simulink model "twintrackSimulinkTest"  (R2023b)
settings: Solver=ode45  StartTime=0.0  StopTime=140  MaxStep=0.01  RelTol=1e-8
libraries: simulink_extras x1, simulink x1
settings Model: PacingRate=9  Creator=eforce  LastModifiedBy=cigla
settings DebuggingCC: UnconnectedInputMsg=warning  UnconnectedOutputMsg=warning  UnconnectedLineMsg=warning
settings ModelReferenceCC: EnableRefExpFcnMdlSchedulingChecks=on
settings RTWCC: DLArmComputeVersion=19.05

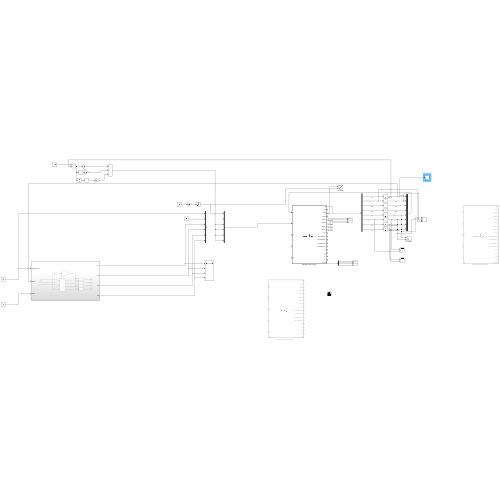
[thumbnail: Simulink's stored preview of the top-level diagram]
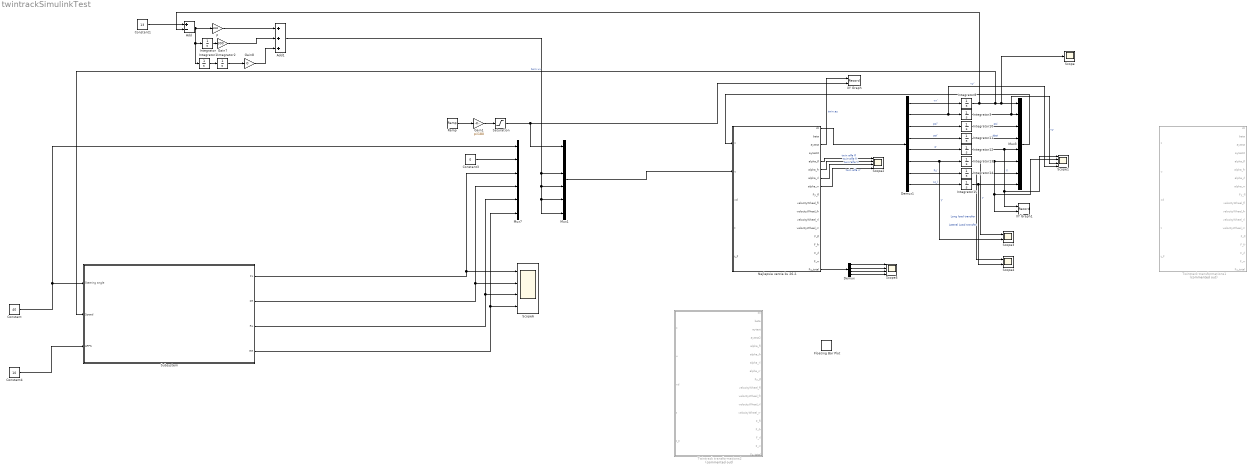
== system twintrackSimulinkTest ==
  Add : Sum  Inputs=+-
  Add1 : Sum  Inputs=+++
  Constant : Constant  Value=40
  Constant1 : Constant  Value=13
  Constant3 : Constant  Value=0
  Constant4 : Constant  Value=10
  Demux : Demux
  Demux1 : Demux  Outputs=8
  Floating Bar Plot : simulink_extras/Additional Sinks/Floating Bar Plot  yLim="[-100 100  -100 100  -100 100  -100 100  -5 5  -5 5  -5 5  -5 5  -5 5  -5 5  -5 5]"
  Gain1 : Gain  Gain=pi/180
  Gain7 : Gain  Gain=300
  Gain8 : Gain  Gain=0
  Integrator{,1..2,8,10..15} (10 alike) : Integrator
  Integrator3 : Integrator  ZeroCross=off
  Mux1 : Mux  Inputs=6
  Mux3 : Mux  Inputs=8
  Mux7 : Mux  Inputs=6
  Najlepsia verzia ku 26.2. : MATLAB Function  TreatAsAtomicUnit=on
  P : Gain  Gain=1000
  Ramp : simulink/Sources/Ramp  slope=0.1  start=10  InitialOutput=0
  Saturation : Saturate  UpperLimit=25  LowerLimit=-25
  Scope : Scope
  Scope{1..2,5..6} (4 alike) : Scope  NumInputPorts=4
  Scope3 : Scope  NumInputPorts=2
  Scope4 : Scope  NumInputPorts=2
  Subsystem : Subsystem
  Twintrack transformations1 : MATLAB Function  Commented=on  TreatAsAtomicUnit=on
  Twintrack transformations2 : MATLAB Function  Commented=on  TreatAsAtomicUnit=on
  XY Graph : Record  FileSettingsInternal="{\"entries\":[{\"content\":{\"excelSettings\":{\"content\":{},\"type\":\"Streamout.ExcelSettings\"}},\"type\":\"Streamout.FileSettingStorage\",\"uuid\":\"\"}],\"packageUris\":[\"http:\\/\\/schema.mathworks.com\\/mf0\\/streamout_blocks\\/R2020a\"],\"version\":\"1.0\"}"  Layout=[1 1]  SignalsInternal="{\"entries\":[{\"content\":{\"signals\":[{\"content\":{\"blockPath\":[],\"dimensions\":[1],\"domain\":\"\",\"lineColor\":\"#edb120\",\"plots\":[1],\"port\":1,\"sid\":[\"\"],\"signalID\":3270,\"signalName\":\"twin.ay\"},\"type\":\"RecordBlkView.Signal\",\"uuid\":\"\"},{\"content\":{\"blockPath\":[],\"dimensions\":[1],\"domain\":\"\",\"lineColor\":\"#7e2f8e\",\"plots\":[1],\"port\":2,\"sid\":[\"\"],\"signalID\":3274,\"signalName\":\"Saturation\"},\"type\":\"RecordBlkView.Signal\",\"uuid\":\"\"}]},\"type\":\"RecordBlkView.InputSignals\",\"uuid\":\"\"}],\"packageUris\":[\"http:\\/\\/schema.mathworks.com\\/mf0\\/streamout_blocks\\/R2020a\"],\"version\":\"1.0\"}"  VisualizationBindings="{\"xyplotplugin\":{\"info\":[{\"series\":[{\"bindingParametersList\":[{\"parameter\":\"X-Axis\",\"signalID\":3270,\"signalName\":\"twin.ay\"},{\"parameter\":\"Y-Axis\",\"signalID\":3274,\"signalName\":\"Saturation\"}],\"seriesID\":12474}],\"subplotID\":1}]}}"  CompatibilityTag=XY
  XY Graph1 : Record  FileSettingsInternal="{\"entries\":[{\"content\":{\"excelSettings\":{\"content\":{},\"type\":\"Streamout.ExcelSettings\"}},\"type\":\"Streamout.FileSettingStorage\",\"uuid\":\"\"}],\"packageUris\":[\"http:\\/\\/schema.mathworks.com\\/mf0\\/streamout_blocks\\/R2020a\"],\"version\":\"1.0\"}"  Layout=[1 1]  SignalsInternal="{\"entries\":[{\"content\":{\"signals\":[{\"content\":{\"blockPath\":[],\"dimensions\":[1],\"domain\":\"\",\"lineColor\":\"#77ac30\",\"plots\":[1],\"port\":1,\"sid\":[\"\"],\"signalID\":3278,\"signalName\":\"X\"},\"type\":\"RecordBlkView.Signal\",\"uuid\":\"\"},{\"content\":{\"blockPath\":[],\"dimensions\":[1],\"domain\":\"\",\"lineColor\":\"#4dbeee\",\"plots\":[1],\"port\":2,\"sid\":[\"\"],\"signalID\":3282,\"signalName\":\"Y\"},\"type\":\"RecordBlkView.Signal\",\"uuid\":\"\"}]},\"type\":\"RecordBlkView.InputSignals\",\"uuid\":\"\"}],\"packageUris\":[\"http:\\/\\/schema.mathworks.com\\/mf0\\/streamout_blocks\\/R2020a\"],\"version\":\"1.0\"}"  VisualizationBindings="{\"xyplotplugin\":{\"info\":[{\"series\":[{\"bindingParametersList\":[{\"parameter\":\"X-Axis\",\"signalID\":3278,\"signalName\":\"X\"},{\"parameter\":\"Y-Axis\",\"signalID\":3282,\"signalName\":\"Y\"}],\"seriesID\":46744}],\"subplotID\":1}]}}"  CompatibilityTag=XY
  wires:
  Constant3/1 -> Mux7/2
  Constant1/1 -> Add/1
  Integrator2/1 -> Gain8/1
  Integrator1/1 -> Integrator2/1
  Mux1/1 -> Najlepsia verzia ku 26.2./2(u)
  Gain7/1 -> Add1/2
  Gain8/1 -> Add1/3
  P/1 -> Add1/1
  Add/1 -> P/1, Integrator/1, Integrator1/1
  Integrator/1 -> Gain7/1
  Integrator8/1 -> Subsystem/2(Speed), Scope/1, Mux3/1, Add/2  "twin.vx"
  Demux1/4 -> Integrator11/1  "psi'"
  Integrator13/1 -> Scope3/1, XY Graph1/2, Scope1/2, Mux3/6  "Y"
  Integrator10/1 -> Mux3/3  "psi"
  Demux1/1 -> Integrator8/1  "vx'"
  Demux1/6 -> Scope3/2, Integrator13/1  "Y'"
  Integrator3/1 -> Scope1/3, Mux3/2  "vy"
  Demux1/7 -> Integrator14/1  "Fz'"
  Demux1/3 -> Integrator10/1  "psi''"
  Demux1/2 -> Scope1/4, Integrator3/1  "vy'"
  Integrator11/1 -> Mux3/4  "dpsi"
  Demux1/5 -> Integrator12/1  "X'"
  Integrator12/1 -> XY Graph1/1, Scope1/1, Mux3/5  "X"
  Demux1/8 -> Integrator15/1  "Lt_l"
  Integrator15/1 -> Scope4/2, Mux3/8  "Lateral Load transfer"
  Integrator14/1 -> Scope4/1, Mux3/7  "Long load transfer"
  Najlepsia verzia ku 26.2./1(dz) -> Demux1/1
  Najlepsia verzia ku 26.2./3(aytest) -> XY Graph/1  "twin.ay"
  Mux3/1 -> Najlepsia verzia ku 26.2./1(z)
  Saturation/1 -> XY Graph/2, Mux1/1
  Najlepsia verzia ku 26.2./18(Fz_total) -> Demux/1
  Demux/1 -> Scope5/1
  Demux/2 -> Scope5/2
  Demux/3 -> Scope5/3
  Demux/4 -> Scope5/4
  Constant/1 -> Mux7/1, Subsystem/1(Steering angle)
  Constant4/1 -> Subsystem/3(APPS)
  Subsystem/1(FL) -> Mux7/3, Scope6/1
  Subsystem/2(FR) -> Scope6/2, Mux7/4
  Subsystem/3(RL) -> Mux7/5, Scope6/3
  Subsystem/4(RR) -> Mux7/6, Scope6/4
  Add1/1 -> Mux1/6, Mux1/5, Mux1/4, Mux1/3
  Ramp/1 -> Gain1/1
  Gain1/1 -> Saturation/1
  Najlepsia verzia ku 26.2./5(alpha_fl) -> Scope2/1  "twin alfa fl"
  Najlepsia verzia ku 26.2./6(alpha_fr) -> Scope2/2  "twin alfa fr"
  Najlepsia verzia ku 26.2./7(alpha_rl) -> Scope2/3  "twin alfa rl"
  Najlepsia verzia ku 26.2./8(alpha_rr) -> Scope2/4  "twin alfa rr"

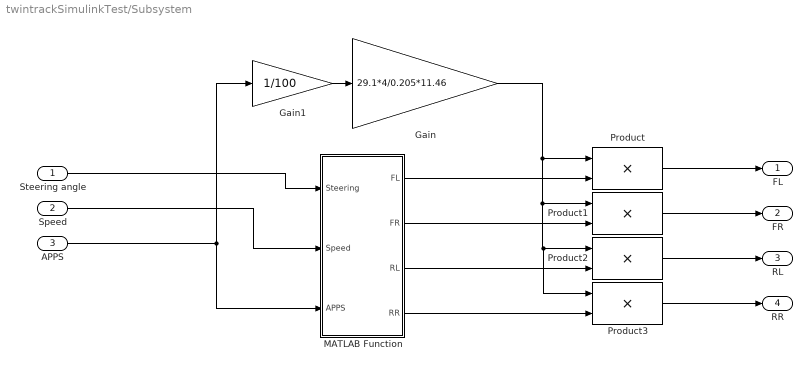
== system twintrackSimulinkTest/Subsystem ==
  Steering angle : Inport
  Speed : Inport  Port=2
  APPS : Inport  Port=3
  Gain : Gain  Gain=29.1*4/0.205*11.46
  Gain1 : Gain  Gain=1/100
  MATLAB Function : MATLAB Function  TreatAsAtomicUnit=on
  Product{,1..3} (4 alike) : Product
  FL : Outport
  FR : Outport  Port=2
  RL : Outport  Port=3
  RR : Outport  Port=4
  wires:
  Steering angle/1 -> MATLAB Function/1(Steering)
  Speed/1 -> MATLAB Function/2(Speed)
  APPS/1 -> Gain1/1, MATLAB Function/3(APPS)
  Gain1/1 -> Gain/1
  MATLAB Function/1(FL) -> Product/2
  Gain/1 -> Product3/1, Product2/1, Product1/1, Product/1
  MATLAB Function/2(FR) -> Product1/2
  MATLAB Function/3(RL) -> Product2/2
  MATLAB Function/4(RR) -> Product3/2
  Product/1 -> FL/1
  Product1/1 -> FR/1
  Product2/1 -> RL/1
  Product3/1 -> RR/1

== matlab function twintrackSimulinkTest/Twintrack transformations2 ==
  data: z input size=8; u input size=6; dz output size=8; xd input; t input; t_F input; beta output; aytest output; aytest2 output; alpha_fl output; alpha_fr output; alpha_rl output; alpha_rr output; Fy_fl output; velocityWheel_fl output size=[1 3]; velocityWheel_fr output size=[1 3]; velocityWheel_rl output size=[1 3]; velocityWheel_rr output size=[1 3]; F_fl output size=[1 2]; F_fr output size=[1 2]; F_rl output size=[1 2]; F_rr output size=[1 2]; Fz_total output size=[1 4]
function [dz, beta, aytest, aytest2,alpha_fl,alpha_fr,alpha_rl,alpha_rr,Fy_fl,velocityWheel_fl,velocityWheel_fr,velocityWheel_rl,velocityWheel_rr,F_fl,F_fr,F_rl,F_rr,Fz_total]= twinRaceCar_time_ODE(z, u, xd, t, t_F)
% z = [vx; vy; psi; dpsidt; X; Y], vx-longitudinal velocity, vy-lateral velocity, psi-angular position of the car with respect to the inertial frame, X and Y are coordinates of the car in the inertial frame
% u = [delta_f; delta_r; Ff; Fr], delta_f - steering angle of the front wheel, delta_r - steering angle of the rear wheel (NOT IMPLEMENTED YET), Ff - force acting on the front wheel in the longitudinal direction, Fr - force acting on the rear wheel in the longitudinal direction
% car - structure containing parameters of the car model




%%%%%%%%%%%%%%%%%%%% Car parameters %%%%%%%%%%%%%%%%%%%%
tracks       = 2;
m            = 280;                      % weight of the car [kg]
Izz          = 100;                      % moment of inertia [kg m^2]
wheelbase    = 1.530;%1.575;                    % distance between the front and rear axles [m];
track        = 1*1.2;                      % distance between right and left wheel
COGr         = 0.4876;                       % COG distribution 0-1 scale on rear
COG          = wheelbase*(COGr); % distance of Center Of Gravity (COG) from the front axle [m];
l_f          = COG;                  % distance of the front axle form the COG [m];
l_r          = wheelbase - COG;  % distance of the rear axle form the COG [m];
COGz         = 0.3;                      % height of COG from ground
wheelradius  = 0.205;                    % radius of the wheels [m]
steeringAngle_max = 20/180*pi;           % Maximum allowed steering angle
steeringAngle_maxRate = 400/180*pi;      % Maximum allowed steering angle [rad/s]
%% Motor parameters
Mf_max       = 29.1 * 2/tracks * 11.46;         % maximum torque generated by a motor on the front axle [Nm]
Mf_slewRate  = 16000;                      % maximum slew rate of the generated torque on the rear axle [Nm/s]0.5 je ca 1000/s idk preco
Mf_jerk       = 800;                           % 1000 bolo cca okay
Mr_max       = 29.1 * 2/tracks * 11.46;         % maximum torque generated by a motor on the rear axle [Nm]
Mr_slewRate  = 100;                      % maximum slew rate of the generated torque on the rear axle [Nm/s]
Yt_max       = (Mf_max/wheelradius + Mr_max/wheelradius)*track;                    % maximum Yaw moment
PwrMax       = 80000;
PwrMin       = -40000;
maxSpeed     = 40;                        %m/sftire


%% Tire and suspension parameters
E = 0.23;
D = 1.2;
B = 0.2;
C = 1.3;


Sus_t = 10;                          % suspension time constant for 1st order system
tire_fxFactor = 1.5 ;                 % max Fx = Fz * tire_fxFactor
tire_fyFactor = 1.3;                 % max Fy = Fz * tire_fyFactor
%ftire = @(alph, Fz, p)(alph/pi*180)* Fz * tire_stifness ; %
ftire = @(alph,Fz, p)  Fz* D*sin(C*atan(B*(alph/pi*180)  - E*atan(B*(alph/pi*180))));
ftire = @(alph, Fz)(alph./pi.*180)./3.* Fz .* tire_fyFactor ; %
%ftire = @(alph, Fz) min((alph./pi.*180)./15.* Fz .* tire_fyFactor ,(deg2rad(15)./pi.*180)./15.* Fz.* tire_fyFactor ) ; %
%% Aerodynamics parameters
CL  = -4.15;
CD  = 1.55;
A   = 1;
COP = 0.5;    % Center of pressure on rear ratio
wingLength_f = 0.9;

%% environment parameters
g = 9.81;
airDensity = 1.225;


    Ft = u;

% Extract the controls from F
delta_f   = Ft(1);
delta_r   = Ft(2);
Fx_fl     = Ft(3);
Fx_fr     = Ft(4);
Fx_rl     = Ft(5);
Fx_rr     = Ft(6);


%% Extract the states from z
v_x  = z(1);
v_y  = z(2);
psi  = z(3);
dpsi = z(4);
X    = z(5);
Y    = z(6);
Fz   = z(7);
Ltl  = z(8);
%% Compute the slip angles
%% Compute the slip angles
%% initialize matrices, origin of car is in COG
v = [v_x v_y 0];
dpsiv = [ 0 0 dpsi];
pos_fr = [  l_f  -track/2 0];
pos_fl = [  l_f   track/2 0];
pos_rr = [ -l_r -track/2 0];
pos_rl = [ -l_r  track/2 0];

%% Calculate vectors at uprights
velocityUpright_fl = v + cross(dpsiv,pos_fl);
velocityUpright_fr = v + cross(dpsiv,pos_fr);
velocityUpright_rl = v + cross(dpsiv,pos_rl);
velocityUpright_rr = v + cross(dpsiv,pos_rr);

%% Define Rotation matrices
rotate_f = [
    cos(delta_f) -sin(delta_f) 0
    sin(delta_f) cos(delta_f)  0
    0            0             0
    ];
rotate_r = [
    cos(delta_r) -sin(delta_r) 0
    sin(delta_r) cos(delta_r)  0
    0            0             0
    ];

%% Calculate wheel velocity in wheel frames
velocityWheel_fl = velocityUpright_fl * rotate_f;
velocityWheel_fr = velocityUpright_fr * rotate_f;
velocityWheel_rl = velocityUpright_rl * rotate_r;
velocityWheel_rr = velocityUpright_rr * rotate_r;


%% Calculate alphas
alpha_fl = -atan2(velocityWheel_fl(2),velocityWheel_fl(1));
alpha_fr = -atan2(velocityWheel_fr(2),velocityWheel_fr(1));
alpha_rl = -atan2(velocityWheel_rl(2),velocityWheel_rl(1));
alpha_rr = -atan2(velocityWheel_rr(2),velocityWheel_rr(1));


%% Compute the forces acting on the wheels
Fz_aero = 0.5*airDensity*CL*A*v_x.^2;
Fz_f = m/2*(1-COGr) * g - Fz/2 - Fz_aero/2 * (1-COP);
Fz_r = m/2*(COGr)   * g + Fz/2 - Fz_aero/2 * COP;

Fz_fl = m/2*(1-COGr) * g - Fz/2 - Fz_aero/2 * (1-COP) + Ltl/2;
Fz_fr = m/2*(1-COGr) * g - Fz/2 - Fz_aero/2 * (1-COP) - Ltl/2;
Fz_rl = m/2*(COGr)   * g + Fz/2 - Fz_aero/2 * COP + Ltl/2;
Fz_rr = m/2*(COGr)   * g + Fz/2 - Fz_aero/2 * COP - Ltl/2;

Fy_fl = ftire(alpha_fl,Fz_fl);
Fy_fr = ftire(alpha_fr,Fz_fr);
Fy_rl = ftire(alpha_rl,Fz_rl);
Fy_rr = ftire(alpha_rr,Fz_rr);

%% Projection of forces from steered wheels to uprights
projection_f = [
    cos(delta_f)      sin(delta_f)
    -sin(delta_f)     cos(delta_f)   
    ];
projection_r = [
    cos(delta_r)      sin(delta_r)
    -sin(delta_r)     cos(delta_r)   
    ];
%% Forces acting on uprights
F_fl = [Fx_fl Fy_fl] * projection_f;
F_fr = [Fx_fr Fy_fr] * projection_f;
F_rl = [Fx_rl Fy_rl] * projection_r;
F_rr = [Fx_rr Fy_rr] * projection_r;

F_drag = 0.5*airDensity*CD*A*v_x^2;
% Compute quantities need for the change of the position in the inertial frame
v = sqrt(v_x^2 + v_y^2);
beta = atan2(v_y, v_x);

M = (F_fr(1) + F_rr(1) - F_fl(1) - F_rl(1))*track/2 +... % Forward forces create Moment
    (F_fr(2) + F_fl(2)) * l_f...                         % Lateral forces from front tires
   -(F_rr(2) + F_rl(2)) * l_r;                          % Lateral forces from rear tires

Fx = F_fr(1) + F_rr(1) + F_fl(1) + F_rl(1)- F_drag;         % Longitudinal force from wheels and drag
Fy = F_fr(2) + F_rr(2) + F_fl(2) + F_rl(2);                  % Lateral force
aytest = Fy/m;
aytest2 = -dpsi*v_x;
Fz_total = [Fz_fl Fz_fr Fz_rl Fz_rr];
%dvx = 1/m  * (F_rx*cos(delta_r) - F_ry*sin(delta_r) + F_fx*cos(delta_f) - F_fy*sin(delta_f) - 0.5*airDensity*CD*A*v_x^2) + dpsi*v_y;
dz = [... 
Fx/m  + dpsi*v_y                                                                                                                      % v_x/dt
Fy/m  - dpsi*v_x                      % v_y/dt  
dpsi;                                                                                                                         % psi/dt
M/Izz   % dpsi
v*cos(psi + beta);                                                                                                            % X/dt
v*sin(psi + beta);                                                                                                            % Y/dt
((Fx/m + dpsi*v_y) *COGz/wheelbase*m-Fz)/Sus_t;                                                                              %Fz/dt  
((- dpsi*v_x) *COGz/track*m-Ltl)/Sus_t;
];

M=4;
end

== matlab function twintrackSimulinkTest/Twintrack transformations1 ==
  data: z input size=8; u input size=6; dz output size=8; xd input; t input; t_F input; beta output; aytest output; aytest2 output; alpha_fl output; alpha_fr output; alpha_rl output; alpha_rr output; Fy_fl output; velocityWheel_fl output size=[1 3]; velocityWheel_fr output size=[1 3]; velocityWheel_rl output size=[1 3]; velocityWheel_rr output size=[1 3]; F_fl output size=[1 2]; F_fr output size=[1 2]; F_rl output size=[1 2]; F_rr output size=[1 2]; Fz_total output size=[1 4]
function [dz, beta, aytest, aytest2,alpha_fl,alpha_fr,alpha_rl,alpha_rr,Fy_fl,velocityWheel_fl,velocityWheel_fr,velocityWheel_rl,velocityWheel_rr,F_fl,F_fr,F_rl,F_rr,Fz_total]= twinRaceCar_time_ODE(z, u, xd, t, t_F)
% z = [vx; vy; psi; dpsidt; X; Y], vx-longitudinal velocity, vy-lateral velocity, psi-angular position of the car with respect to the inertial frame, X and Y are coordinates of the car in the inertial frame
% u = [delta_f; delta_r; Ff; Fr], delta_f - steering angle of the front wheel, delta_r - steering angle of the rear wheel (NOT IMPLEMENTED YET), Ff - force acting on the front wheel in the longitudinal direction, Fr - force acting on the rear wheel in the longitudinal direction
% car - structure containing parameters of the car model




%%%%%%%%%%%%%%%%%%%% Car parameters %%%%%%%%%%%%%%%%%%%%
tracks       = 2;
m            = 280;                      % weight of the car [kg]
Izz          = 100;                      % moment of inertia [kg m^2]
wheelbase    = 1.530;%1.575;                    % distance between the front and rear axles [m];
track        = 1*1.2;                      % distance between right and left wheel
COGr         = 0.4876;                       % COG distribution 0-1 scale on rear
COG          = wheelbase*(COGr); % distance of Center Of Gravity (COG) from the front axle [m];
l_f          = COG;                  % distance of the front axle form the COG [m];
l_r          = wheelbase - COG;  % distance of the rear axle form the COG [m];
COGz         = 0.3;                      % height of COG from ground
wheelradius  = 0.205;                    % radius of the wheels [m]
steeringAngle_max = 20/180*pi;           % Maximum allowed steering angle
steeringAngle_maxRate = 400/180*pi;      % Maximum allowed steering angle [rad/s]
%% Motor parameters
Mf_max       = 29.1 * 2/tracks * 11.46;         % maximum torque generated by a motor on the front axle [Nm]
Mf_slewRate  = 16000;                      % maximum slew rate of the generated torque on the rear axle [Nm/s]0.5 je ca 1000/s idk preco
Mf_jerk       = 800;                           % 1000 bolo cca okay
Mr_max       = 29.1 * 2/tracks * 11.46;         % maximum torque generated by a motor on the rear axle [Nm]
Mr_slewRate  = 100;                      % maximum slew rate of the generated torque on the rear axle [Nm/s]
Yt_max       = (Mf_max/wheelradius + Mr_max/wheelradius)*track;                    % maximum Yaw moment
PwrMax       = 80000;
PwrMin       = -40000;
maxSpeed     = 40;                        %m/sftire


%% Tire and suspension parameters
E = 0.23;
D = 1.2;
B = 0.2;
C = 1.3;


Sus_t = 10;                          % suspension time constant for 1st order system
tire_fxFactor = 1.5 ;                 % max Fx = Fz * tire_fxFactor
tire_fyFactor = 1.3;                 % max Fy = Fz * tire_fyFactor
%ftire = @(alph, Fz, p)(alph/pi*180)* Fz * tire_stifness ; %
ftire = @(alph,Fz, p)  Fz* D*sin(C*atan(B*(alph/pi*180)  - E*atan(B*(alph/pi*180))));
%ftire = @(alph, Fz)(alph./pi.*180)./3.* Fz .* tire_fyFactor ; %
%ftire = @(alph, Fz) min((alph./pi.*180)./15.* Fz .* tire_fyFactor ,(deg2rad(15)./pi.*180)./15.* Fz.* tire_fyFactor ) ; %
%% Aerodynamics parameters
CL  = -4.15;
CD  = 1.55;
A   = 1;
COP = 0.5;    % Center of pressure on rear ratio
wingLength_f = 0.9;

%% environment parameters
g = 9.81;
airDensity = 1.225;


    Ft = u;

% Extract the controls from F
delta_f   = Ft(1);
delta_r   = Ft(2);
Fx_fl     = Ft(3);
Fx_fr     = Ft(4);
Fx_rl     = Ft(5);
Fx_rr     = Ft(6);


%% Extract the states from z
v_x  = z(1);
v_y  = z(2);
psi  = z(3);
dpsi = z(4);
X    = z(5);
Y    = z(6);
Fz   = z(7);
Ltl  = z(8);
%% Compute the slip angles
%% Compute the slip angles
%% initialize matrices, origin of car is in COG
v = [v_x v_y 0];
dpsiv = [ 0 0 dpsi];
pos_fr = [  l_f  -track/2 0];
pos_fl = [  l_f   track/2 0];
pos_rr = [ -l_r -track/2 0];
pos_rl = [ -l_r  track/2 0];

%% Calculate vectors at uprights
velocityUpright_fl = v + cross(dpsiv,pos_fl);
velocityUpright_fr = v + cross(dpsiv,pos_fr);
velocityUpright_rl = v + cross(dpsiv,pos_rl);
velocityUpright_rr = v + cross(dpsiv,pos_rr);

%% Define Rotation matrices
rotate_f = [
    cos(delta_f) -sin(delta_f) 0
    sin(delta_f) cos(delta_f)  0
    0            0             0
    ];
rotate_r = [
    cos(delta_r) -sin(delta_r) 0
    sin(delta_r) cos(delta_r)  0
    0            0             0
    ];

%% Calculate wheel velocity in wheel frames
velocityWheel_fl = velocityUpright_fl * rotate_f;
velocityWheel_fr = velocityUpright_fr * rotate_f;
velocityWheel_rl = velocityUpright_rl * rotate_r;
velocityWheel_rr = velocityUpright_rr * rotate_r;


%% Calculate alphas
alpha_fl = -atan2(velocityWheel_fl(2),velocityWheel_fl(1));
alpha_fr = -atan2(velocityWheel_fr(2),velocityWheel_fr(1));
alpha_rl = -atan2(velocityWheel_rl(2),velocityWheel_rl(1));
alpha_rr = -atan2(velocityWheel_rr(2),velocityWheel_rr(1));


%% Compute the forces acting on the wheels
Fz_aero = 0.5*airDensity*CL*A*v_x.^2;
Fz_f = m/2*(1-COGr) * g - Fz/2 - Fz_aero/2 * (1-COP);
Fz_r = m/2*(COGr)   * g + Fz/2 - Fz_aero/2 * COP;

Fz_fl = m/2*(1-COGr) * g - Fz/2 - Fz_aero/2 * (1-COP) + Ltl/2;
Fz_fr = m/2*(1-COGr) * g - Fz/2 - Fz_aero/2 * (1-COP) - Ltl/2;
Fz_rl = m/2*(COGr)   * g + Fz/2 - Fz_aero/2 * COP + Ltl/2;
Fz_rr = m/2*(COGr)   * g + Fz/2 - Fz_aero/2 * COP - Ltl/2;

Fz_total = [Fz_fl Fz_fr Fz_rl Fz_rr];

Fy_fl = ftire(alpha_fl,Fz_fl);
Fy_fr = ftire(alpha_fr,Fz_fr);
Fy_rl = ftire(alpha_rl,Fz_rl);
Fy_rr = ftire(alpha_rr,Fz_rr);

%% Projection of forces from steered wheels to uprights
projection_f = [
    cos(delta_f)      sin(delta_f)
    -sin(delta_f)     cos(delta_f)   
    ];

%projection_f = [
%    -cos(delta_f)      sin(delta_f)
%    sin(delta_f)     cos(delta_f)   
%    ];

projection_r = [
    cos(delta_r)      sin(delta_r)
    -sin(delta_r)     cos(delta_r)   
    ];
%% Forces acting on uprights
F_fl = [Fx_fl Fy_fl] * projection_f;
F_fr = [Fx_fr Fy_fr] * projection_f;
F_rl = [Fx_rl Fy_rl] * projection_r;
F_rr = [Fx_rr Fy_rr] * projection_r;

F_drag = 0.5*airDensity*CD*A*v_x^2;
% Compute quantities need for the change of the position in the inertial frame
v = sqrt(v_x^2 + v_y^2);
beta = atan2(v_y, v_x);

M = (F_fr(1) + F_rr(1) - F_fl(1) - F_rl(1))*track/2 +... % Forward forces create Moment
    (F_fr(2) + F_fl(2)) * l_f...                         % Lateral forces from front tires
   -(F_rr(2) + F_rl(2)) * l_r;                          % Lateral forces from rear tires

Fx = F_fr(1) + F_rr(1) + F_fl(1) + F_rl(1)- F_drag;         % Longitudinal force from wheels and drag
Fy = F_fr(2) + F_rr(2) + F_fl(2) + F_rl(2);                  % Lateral force

aytest = Fy/m;
aytest2 = -dpsi*v_x;

%dvx = 1/m  * (F_rx*cos(delta_r) - F_ry*sin(delta_r) + F_fx*cos(delta_f) - F_fy*sin(delta_f) - 0.5*airDensity*CD*A*v_x^2) + dpsi*v_y;
dz = [... 
Fx/m  + dpsi*v_y                                                                                                                      % v_x/dt
Fy/m  - dpsi*v_x                      % v_y/dt  
dpsi;                                                                                                                         % psi/dt
M/Izz   % dpsi
v*cos(psi + beta);                                                                                                            % X/dt
v*sin(psi + beta);                                                                                                            % Y/dt
((Fx/m + dpsi*v_y) *COGz/wheelbase*m-Fz)/Sus_t;                                                                              %Fz/dt  
((- dpsi*v_x) *COGz/track*m-Ltl)/Sus_t;
];

M=4;
end

== matlab function twintrackSimulinkTest/Subsystem/MATLAB Function ==
  data: Steering input; FL output; Speed input; APPS input; FR output; RL output; RR output
function [FL,FR,RL,RR] = fcn(Steering, Speed, APPS)

kL = 0.4;
k1 = 10;
kS = 0.75;

Steer_cal =Steering-50;
Mz = APPS*kL-Speed*(kL*APPS/33)+50+k1;
Ms = Steer_cal*kS-Speed*(kS*Steer_cal/33);



FL = 50-(Mz/2)+(Ms/2);
FR = 50-(Mz/2)-(Ms/2);

RL  =Mz/2+(Ms/2); 
RR  =(Mz/2)-(Ms/2);

== matlab function twintrackSimulinkTest/Najlepsia verzia ku 26.2. ==
  data: z input size=8; u input size=6; dz output size=8; xd input; t input; t_F input; beta output; aytest output; aytest2 output; alpha_fl output; alpha_fr output; alpha_rl output; alpha_rr output; Fy_fl output; velocityWheel_fl output size=[1 3]; velocityWheel_fr output size=[1 3]; velocityWheel_rl output size=[1 3]; velocityWheel_rr output size=[1 3]; F_fl output size=[1 2]; F_fr output size=[1 2]; F_rl output size=[1 2]; F_rr output size=[1 2]; Fz_total output size=[1 4]
function [dz, beta, aytest, aytest2,alpha_fl,alpha_fr,alpha_rl,alpha_rr,Fy_fl,velocityWheel_fl,velocityWheel_fr,velocityWheel_rl,velocityWheel_rr,F_fl,F_fr,F_rl,F_rr,Fz_total]= twinRaceCar_time_ODE(z, u, xd, t, t_F)
% z = [vx; vy; psi; dpsidt; X; Y], vx-longitudinal velocity, vy-lateral velocity, psi-angular position of the car with respect to the inertial frame, X and Y are coordinates of the car in the inertial frame
% u = [delta_f; delta_r; Ff; Fr], delta_f - steering angle of the front wheel, delta_r - steering angle of the rear wheel (NOT IMPLEMENTED YET), Ff - force acting on the front wheel in the longitudinal direction, Fr - force acting on the rear wheel in the longitudinal direction
% car - structure containing parameters of the car model




%%%%%%%%%%%%%%%%%%%% Car parameters %%%%%%%%%%%%%%%%%%%%
tracks       = 2;
m            = 280;                      % weight of the car [kg]
Izz          = 100;                      % moment of inertia [kg m^2]
wheelbase    = 1.530;%1.575;                    % distance between the front and rear axles [m];
track        = 1*1.2;                      % distance between right and left wheel
COGr         = 0.4876;                       % COG distribution 0-1 scale on rear
COG          = wheelbase*(COGr); % distance of Center Of Gravity (COG) from the front axle [m];
l_f          = COG;                  % distance of the front axle form the COG [m];
l_r          = wheelbase - COG;  % distance of the rear axle form the COG [m];
COGz         = 0.3;                      % height of COG from ground
wheelradius  = 0.205;                    % radius of the wheels [m]
steeringAngle_max = 20/180*pi;           % Maximum allowed steering angle
steeringAngle_maxRate = 400/180*pi;      % Maximum allowed steering angle [rad/s]
%% Motor parameters
Mf_max       = 29.1 * 2/tracks * 11.46;         % maximum torque generated by a motor on the front axle [Nm]
Mf_slewRate  = 16000;                      % maximum slew rate of the generated torque on the rear axle [Nm/s]0.5 je ca 1000/s idk preco
Mf_jerk       = 800;                           % 1000 bolo cca okay
Mr_max       = 29.1 * 2/tracks * 11.46;         % maximum torque generated by a motor on the rear axle [Nm]
Mr_slewRate  = 100;                      % maximum slew rate of the generated torque on the rear axle [Nm/s]
Yt_max       = (Mf_max/wheelradius + Mr_max/wheelradius)*track;                    % maximum Yaw moment
PwrMax       = 80000;
PwrMin       = -40000;
maxSpeed     = 40;                        %m/sftire


%% Tire and suspension parameters
E = 0.23;
D = 1.2;
B = 0.2;
C = 1.3;


Sus_t = 0.05;                          % suspension time constant for 1st order system
tire_fxFactor = 1.5 ;                 % max Fx = Fz * tire_fxFactor
tire_fyFactor = 1.3;                 % max Fy = Fz * tire_fyFactor
%ftire = @(alph, Fz, p)(alph/pi*180)* Fz * tire_stifness ; %
ftire = @(alph,Fz, p)  Fz* D*sin(C*atan(B*(alph/pi*180)  - E*atan(B*(alph/pi*180))));
ftire = @(alph, Fz)(alph./pi.*180)./3.* Fz .* tire_fyFactor ; %
%ftire = @(alph, Fz) min((alph./pi.*180)./15.* Fz .* tire_fyFactor ,(deg2rad(15)./pi.*180)./15.* Fz.* tire_fyFactor ) ; %
%% Aerodynamics parameters
CL  = -4.15;
CD  = 1.55;
A   = 1;
COP = 0.5;    % Center of pressure on rear ratio
wingLength_f = 0.9;

%% environment parameters
g = 9.81;
airDensity = 1.225;


    Ft = u;

% Extract the controls from F
delta_f   = Ft(1);
delta_r   = Ft(2);
Fx_fl     = Ft(3);
Fx_fr     = Ft(4);
Fx_rl     = Ft(5);
Fx_rr     = Ft(6);


%% Extract the states from z
v_x  = z(1);
v_y  = z(2);
psi  = z(3);
dpsi = z(4);
X    = z(5);
Y    = z(6);
Fz   = z(7);
Ltl  = z(8);
%% Compute the slip angles
%% Compute the slip angles
%% initialize matrices, origin of car is in COG
v = [v_x v_y 0];
dpsiv = [ 0 0 dpsi];
pos_fr = [  l_f  -track/2 0];
pos_fl = [  l_f   track/2 0];
pos_rr = [ -l_r -track/2 0];
pos_rl = [ -l_r  track/2 0];

%% Calculate vectors at uprights
velocityUpright_fl = v + cross(dpsiv,pos_fl);
velocityUpright_fr = v + cross(dpsiv,pos_fr);
velocityUpright_rl = v + cross(dpsiv,pos_rl);
velocityUpright_rr = v + cross(dpsiv,pos_rr);

%% Define Rotation matrices
rotate_f = [
    cos(delta_f) -sin(delta_f) 0
    sin(delta_f) cos(delta_f)  0
    0            0             0
    ];
rotate_r = [
    cos(delta_r) -sin(delta_r) 0
    sin(delta_r) cos(delta_r)  0
    0            0             0
    ];

%% Calculate wheel velocity in wheel frames
velocityWheel_fl = velocityUpright_fl * rotate_f;
velocityWheel_fr = velocityUpright_fr * rotate_f;
velocityWheel_rl = velocityUpright_rl * rotate_r;
velocityWheel_rr = velocityUpright_rr * rotate_r;


%% Calculate alphas
alpha_fl = -atan2(velocityWheel_fl(2),velocityWheel_fl(1));
alpha_fr = -atan2(velocityWheel_fr(2),velocityWheel_fr(1));
alpha_rl = -atan2(velocityWheel_rl(2),velocityWheel_rl(1));
alpha_rr = -atan2(velocityWheel_rr(2),velocityWheel_rr(1));


%% Compute the forces acting on the wheels
Fz_aero = 0.5*airDensity*CL*A*v_x.^2;
Fz_f = m/2*(1-COGr) * g - Fz/2 - Fz_aero/2 * (1-COP);
Fz_r = m/2*(COGr)   * g + Fz/2 - Fz_aero/2 * COP;

Fz_fl = m/2*(1-COGr) * g - Fz/2 - Fz_aero/2 * (1-COP) - Ltl/2;
Fz_fr = m/2*(1-COGr) * g - Fz/2 - Fz_aero/2 * (1-COP) + Ltl/2;
Fz_rl = m/2*(COGr)   * g + Fz/2 - Fz_aero/2 * COP - Ltl/2;
Fz_rr = m/2*(COGr)   * g + Fz/2 - Fz_aero/2 * COP + Ltl/2;

Fz_total = [Fz_fl Fz_fr Fz_rl Fz_rr];

Fy_fl = ftire(alpha_fl,Fz_fl);
Fy_fr = ftire(alpha_fr,Fz_fr);
Fy_rl = ftire(alpha_rl,Fz_rl);
Fy_rr = ftire(alpha_rr,Fz_rr);

%% Projection of forces from steered wheels to uprights
projection_f = [
    cos(delta_f)      sin(delta_f)
    -sin(delta_f)     cos(delta_f)   
    ];

%projection_f = [
%    -cos(delta_f)      sin(delta_f)
%    sin(delta_f)     cos(delta_f)   
%    ];

projection_r = [
    cos(delta_r)      sin(delta_r)
    -sin(delta_r)     cos(delta_r)   
    ];
%% Forces acting on uprights
F_fl = [Fx_fl Fy_fl] * projection_f;
F_fr = [Fx_fr Fy_fr] * projection_f;
F_rl = [Fx_rl Fy_rl] * projection_r;
F_rr = [Fx_rr Fy_rr] * projection_r;

F_drag = 0.5*airDensity*CD*A*v_x^2;
% Compute quantities need for the change of the position in the inertial frame
v = sqrt(v_x^2 + v_y^2);
beta = atan2(v_y, v_x);

M = (F_fr(1) + F_rr(1) - F_fl(1) - F_rl(1))*track/2 +... % Forward forces create Moment
    (F_fr(2) + F_fl(2)) * l_f...                         % Lateral forces from front tires
   -(F_rr(2) + F_rl(2)) * l_r;                          % Lateral forces from rear tires

Fx = F_fr(1) + F_rr(1) + F_fl(1) + F_rl(1)- F_drag;         % Longitudinal force from wheels and drag
Fy = F_fr(2) + F_rr(2) + F_fl(2) + F_rl(2);                  % Lateral force

aytest = Fy/m;
aytest2 = -dpsi*v_x;

%dvx = 1/m  * (F_rx*cos(delta_r) - F_ry*sin(delta_r) + F_fx*cos(delta_f) - F_fy*sin(delta_f) - 0.5*airDensity*CD*A*v_x^2) + dpsi*v_y;
dz = [... 
Fx/m  + dpsi*v_y                                                                                                                      % v_x/dt
Fy/m  - dpsi*v_x                      % v_y/dt  
dpsi;                                                                                                                         % psi/dt
M/Izz   % dpsi
v*cos(psi + beta);                                                                                                            % X/dt
v*sin(psi + beta);                                                                                                            % Y/dt
((Fx/m) *COGz/wheelbase*m-Fz)/Sus_t;                                                                              %Fz/dt  
((Fy/m) *COGz/track*m-Ltl)/Sus_t;
];

M=4;
end
